simulink model "sampleModel2"  (R2021a)
settings: Solver=VariableStepAuto  StartTime=0.0  StopTime=10.0  RelTol=1e-3
undefined symbols (not defined in the file): Newton, Raphson
libraries: simulink x14, simulink_need_slupdate x3
settings Model: Creator=user  LastModifiedBy=user

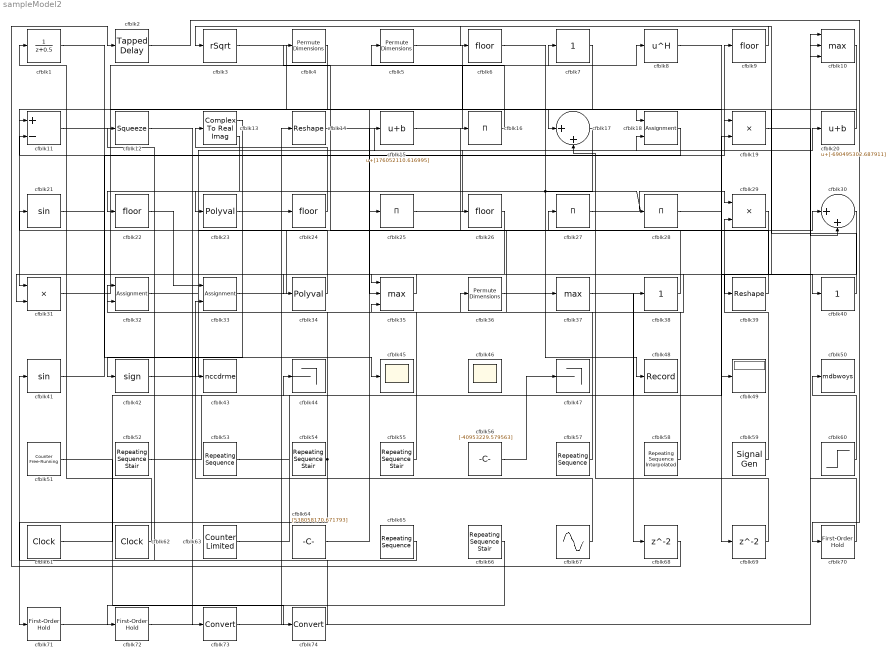
== system sampleModel2 ==
  cfblk1 : DiscreteTransferFcn  SampleTime=1
  cfblk10 : MinMax  Function=max  Inputs=3
  cfblk11 : Sum  Inputs=+-
  cfblk12 : Squeeze
  cfblk13 : ComplexToRealImag
  cfblk14 : Reshape
  cfblk15 : Bias  Bias=[176052110.616995]
  cfblk{16,25,27..28} (4 alike) : Product  Inputs=*
  cfblk17 : Sum  Inputs=|++
  cfblk18 : Assignment  DiagnosticForDimensions=Warning  IndexOptions=Index vector (dialog)  Indices=1  OutputSizes=1
  cfblk19 : Product
  cfblk2 : simulink/Discrete/Tapped Delay  vinit=0.0  samptime=-1  NumDelays=1  DelayOrder=Oldest  includeCurrent=off
  cfblk20 : Bias  Bias=[-690495302.687911]
  cfblk21 : Trigonometry
  cfblk{6,9,22,24,26} (5 alike) : Rounding
  cfblk23 : Polyval  Coefs=[ +2.081618890e-019, -1.441693666e-014, +4.719686976e-010, -8.536869453e-006, +1.621573104e-001, -8.087801117e+001 ]
  cfblk29 : Product
  cfblk3 : Sqrt  Operator=rSqrt  AlgorithmType=Newton-Raphson  SaturateOnIntegerOverflow=on
  cfblk30 : Sum  Inputs=|++
  cfblk31 : Product  Inputs=**
  cfblk32 : Assignment  DiagnosticForDimensions=Warning  IndexOptions=Index vector (dialog)  Indices=1  OutputSizes=1
  cfblk33 : Assignment  DiagnosticForDimensions=Warning  IndexOptions=Index vector (dialog)  Indices=1  OutputSizes=1
  cfblk34 : Polyval  Coefs=[ +2.081618890e-019, -1.441693666e-014, +4.719686976e-010, -8.536869453e-006, +1.621573104e-001, -8.087801117e+001 ]
  cfblk35 : MinMax  Function=max  Inputs=3
  cfblk36 : PermuteDimensions
  cfblk37 : MinMax  Function=max
  cfblk38 : simulink/Math Operations/Slider Gain  gain=1  low=0  high=2
  cfblk39 : Reshape
  cfblk4 : PermuteDimensions
  cfblk40 : simulink/Math Operations/Slider Gain  gain=1  low=0  high=2
  cfblk41 : Trigonometry
  cfblk42 : Signum
  cfblk43 : ToWorkspace  VariableName=nccdrme  SaveFormat=Timeseries  SampleTime=-1
  cfblk44 : Terminator
  cfblk45 : Scope
  cfblk46 : Scope
      settings: Floating=on
  cfblk47 : Terminator
  cfblk48 : Record  FileSettingsInternal="{\"entries\":[{\"content\":{\"excelSettings\":{\"content\":{},\"type\":\"Streamout.ExcelSettings\"}},\"type\":\"Streamout.FileSettingStorage\",\"uuid\":\"24b9c065-b35a-4456-b184-28f1ec945152\"}],\"packageUris\":[\"http://schema.mathworks.com/mf0/streamout_blocks/R2020a\"],\"version\":\"1.0\"}"  SignalsInternal="{\"entries\":[{\"content\":{\"signals\":[{\"content\":{\"blockPath\":[\"sampleModel2/cfblk48\"],\"channel\":[],\"dimensions\":[1,1],\"domain\":\"samplemodel2/cfblk48\",\"lineColor\":\"#22b573\",\"plots\":[1],\"port\":1,\"sid\":[\"\"],\"signalID\":2636780,\"signalName\":\"cfblk36\"},\"type\":\"RecordBlkView.Signal\",\"uuid\":\"599e2e04-604a-4870-9f00-6d08104144b0\"}]},\"type\":\"RecordBlkView.InputSignals\",\"uuid\":\"302f7845-a23d-4261-9b06-e3fc54a68d36\"}],\"packageUris\":[\"http://schema.mathworks.com/mf0/streamout_blocks/R2020a\"],\"version\":\"1.0\"}"  VisualizationBindings="{\"sparklinesplugin\":{\"info\":[{\"bindingParametersList\":[],\"subplotID\":1}]}}"
  cfblk49 : Display
  cfblk5 : PermuteDimensions
  cfblk50 : ToWorkspace  VariableName=mdbwoys  SaveFormat=Timeseries  SampleTime=-1
  cfblk51 : simulink/Sources/Counter Free-Running  NumBits=[35.000000]  tsamp=-1
  cfblk52 : simulink/Sources/Repeating Sequence Stair  OutValues=[630794422.954842, 758027809.194355]  tsamp=-1  OutMin=[]  OutMax=[]  OutDataTypeStr=double  OutputDataTypeScalingMode=double  OutDataType=fixdt(0,8)  ConRadixGroup=Best Precision: Vector-wise  OutScaling=2^-12
  cfblk53 : simulink/Sources/Repeating Sequence  rep_seq_t=[0 2]  rep_seq_y=[977823232.159178, -998955249.286110]
  cfblk54 : simulink/Sources/Repeating Sequence Stair  OutValues=[730877182.026049, 225132938.967998]  tsamp=-1  OutMin=[]  OutMax=[]  OutDataTypeStr=double  OutputDataTypeScalingMode=double  OutDataType=fixdt(0,8)  ConRadixGroup=Best Precision: Vector-wise  OutScaling=2^-12
  cfblk55 : simulink/Sources/Repeating Sequence Stair  OutValues=[979900411.417662, 55360138.676885]  tsamp=-1  OutMin=[]  OutMax=[]  OutDataTypeStr=double  OutputDataTypeScalingMode=double  OutDataType=fixdt(0,8)  ConRadixGroup=Best Precision: Vector-wise  OutScaling=2^-12
  cfblk56 : Constant  Value=[-40953229.579563]  SampleTime=1
  cfblk57 : simulink/Sources/Repeating Sequence  rep_seq_t=[0 2]  rep_seq_y=[-544314128.587916, -3811417.607221]
  cfblk58 : simulink/Sources/Repeating Sequence Interpolated  OutValues=[801704977.064010, 149322438.260375, 690356370.108073, 477280583.990804, 171974071.652952]  TimeValues=[0 0.1 0.5 0.6 1].'  LookUpMeth=Interpolation-Use End Values  tsamp=0.01  OutMin=[]  OutMax=[]  OutDataTypeStr=double  OutputDataTypeScalingMode=double  OutDataType=fixdt(0,8)  OutScaling=2^-10
  cfblk59 : SignalGenerator  Amplitude=[332832434.638936]
  cfblk60 : Step  Time=[33.000000]  Before=[459503710.634442]  After=[781504232.650645]  SampleTime=0
  cfblk61 : DigitalClock
  cfblk62 : DigitalClock
  cfblk63 : simulink/Sources/Counter Limited  uplimit=[982.000000]  tsamp=-1
  cfblk64 : Constant  Value=[538058170.671793]  SampleTime=1
  cfblk65 : simulink/Sources/Repeating Sequence  rep_seq_t=[0 2]  rep_seq_y=[856626124.628376, 160180731.516883]
  cfblk66 : simulink/Sources/Repeating Sequence Stair  OutValues=[-966034123.325477, -758280857.802884]  tsamp=-1  OutMin=[]  OutMax=[]  OutDataTypeStr=double  OutputDataTypeScalingMode=double  OutDataType=fixdt(0,8)  ConRadixGroup=Best Precision: Vector-wise  OutScaling=2^-12
  cfblk67 : Sin  Amplitude=[725421437.399339]  Bias=[-31406977.575795]  SampleTime=0
  cfblk68 : Delay  SampleTime=1
  cfblk69 : Delay  SampleTime=1
  cfblk7 : simulink/Math Operations/Slider Gain  gain=1  low=0  high=2
  cfblk70 : simulink_need_slupdate/First-Order Hold  DisableCoverage=on  Ts=1
      settings: SourceProductBaseCode=SL
  cfblk71 : simulink_need_slupdate/First-Order Hold  DisableCoverage=on  Ts=1
      settings: SourceProductBaseCode=SL
  cfblk72 : simulink_need_slupdate/First-Order Hold  DisableCoverage=on  Ts=1
      settings: SourceProductBaseCode=SL
  cfblk73 : DataTypeConversion
  cfblk74 : DataTypeConversion
  cfblk8 : Math  Operator=hermitian  SaturateOnIntegerOverflow=on
  wires:
  cfblk13/1 -> cfblk42/1
  cfblk38/1 -> cfblk27/1
  cfblk3/1 -> cfblk18/1
  cfblk15/1 -> cfblk7/1
  cfblk14/1 -> cfblk9/1
  cfblk40/1 -> cfblk3/1
  cfblk33/1 -> cfblk16/1
  cfblk29/1 -> cfblk36/1
  cfblk27/1 -> cfblk29/1
  cfblk31/1 -> cfblk8/1
  cfblk61/1 -> cfblk44/1
  cfblk11/1 -> cfblk17/1
  cfblk42/1 -> cfblk30/1
  cfblk13/2 -> cfblk22/1
  cfblk5/1 -> cfblk49/1
  cfblk9/1 -> cfblk6/1
  cfblk4/1 -> cfblk31/1
  cfblk56/1 -> cfblk47/1
  cfblk6/1 -> cfblk37/1, cfblk28/1
  cfblk65/1 -> cfblk41/1
  cfblk60/1 -> cfblk50/1
  cfblk30/1 -> cfblk35/1
  cfblk24/1 -> cfblk13/1
  cfblk21/1 -> cfblk45/1
  cfblk25/1 -> cfblk18/2
  cfblk53/1 -> cfblk25/1
  cfblk62/1 -> cfblk1/1
  cfblk59/1 -> cfblk29/2
  cfblk32/1 -> cfblk20/1
  cfblk16/1 -> cfblk5/1
  cfblk22/1 -> cfblk33/1
  cfblk8/1 -> cfblk40/1
  cfblk36/1 -> cfblk48/1
  cfblk67/1 -> cfblk33/2
  cfblk57/1 -> cfblk26/1
  cfblk7/1 -> cfblk35/2
  cfblk23/1 -> cfblk14/1
  cfblk39/1 -> cfblk4/1
  cfblk17/1 -> cfblk23/1
  cfblk64/1 -> cfblk15/1
  cfblk35/1 -> cfblk34/1
  cfblk10/1 -> cfblk39/1
  cfblk55/1 -> cfblk35/3
  cfblk19/1 -> cfblk30/2
  cfblk26/1 -> cfblk31/2
  cfblk20/1 -> cfblk11/1
  cfblk1/1 -> cfblk43/1
  cfblk18/1 -> cfblk11/2
  cfblk34/1 -> cfblk21/1
  cfblk52/1 -> cfblk38/1
  cfblk54/1 -> cfblk32/2, cfblk71/1
  cfblk41/1 -> cfblk19/1
  cfblk58/1 -> cfblk32/1
  cfblk63/1 -> cfblk19/2
  cfblk37/1 -> cfblk68/1
  cfblk68/1 -> cfblk2/1
  cfblk28/1 -> cfblk69/1
  cfblk69/1 -> cfblk17/2
  cfblk2/1 -> cfblk70/1
  cfblk70/1 -> cfblk10/1
  cfblk71/1 -> cfblk10/2
  cfblk66/1 -> cfblk72/1
  cfblk72/1 -> cfblk10/3
  cfblk12/1 -> cfblk73/1
  cfblk73/1 -> cfblk24/1
  cfblk51/1 -> cfblk74/1
  cfblk74/1 -> cfblk12/1
